simulink model "ClimberRobotModel_rbar_control"  (R2020a)
settings: Solver=VariableStepAuto  StartTime=0.0  StopTime=10.0  RelTol=1e-3
settings Model: Creator=danielefontanelli  LastModifiedBy=danielefontanelli

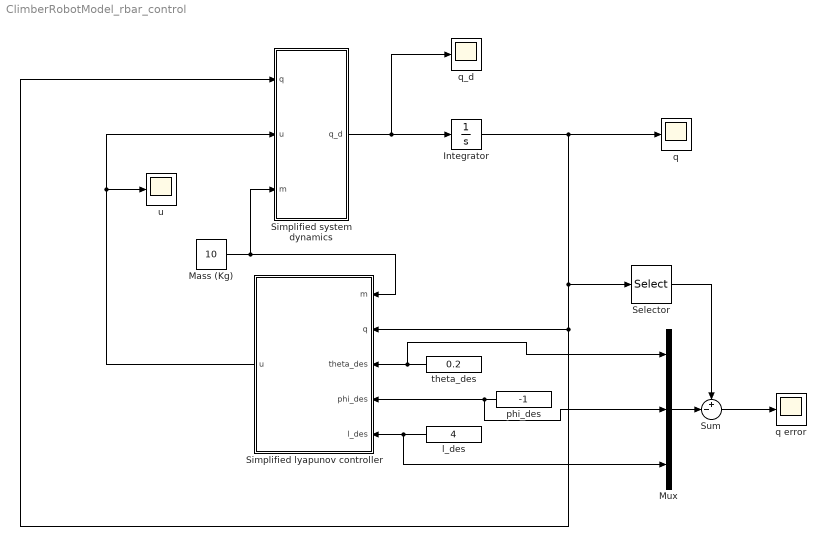
== system ClimberRobotModel_rbar_control ==
  Integrator : Integrator  InitialCondition=[0.2, -0.4, 7, 1, -1, 0]
  Mass (Kg) : Constant  Value=10
  Mux : Mux  Inputs=3
  Selector : Selector  InputPortWidth=6  IndexOptions=Index vector (dialog)  Indices=[1 2 3]  OutputSizes=1
  Simplified lyapunov controller : MATLAB Function  TreatAsAtomicUnit=on
  Simplified system dynamics : MATLAB Function  TreatAsAtomicUnit=on
  Sum : Sum  Inputs=+-|
  l_des : Constant  Value=4
  phi_des : Constant  Value=-1
  q : Scope
  q error : Scope
  q_d : Scope
  theta_des : Constant  Value=0.2
  u : Scope
  wires:
  Mass (Kg)/1 -> Simplified lyapunov controller/1(m), Simplified system dynamics/3(m)
  Simplified system dynamics/1(q_d) -> q_d/1, Integrator/1
  Integrator/1 -> q/1, Simplified system dynamics/1(q), Simplified lyapunov controller/2(q), Selector/1
  Simplified lyapunov controller/1(u) -> u/1, Simplified system dynamics/2(u)
  theta_des/1 -> Mux/1, Simplified lyapunov controller/3(theta_des)
  phi_des/1 -> Mux/2, Simplified lyapunov controller/4(phi_des)
  l_des/1 -> Mux/3, Simplified lyapunov controller/5(l_des)
  Selector/1 -> Sum/1
  Mux/1 -> Sum/2
  Sum/1 -> q error/1

== matlab function ClimberRobotModel_rbar_control/Simplified lyapunov controller ==
  data: m input; q input; u output; theta_des input; phi_des input; l_des input
function u = fcn(m, q, theta_des, phi_des, l_des)

g = 9.8;   % m/s^2

% Gains
k_theta = 1;
k_phi = 1;
k_l = 1;
k_omega = 1;
k_psi = 1;
k_r = 1;

% State space variables
theta = q(1);
phi = q(2);
l = q(3);
omega = q(4);
psi = q(5);
r = q(6);

if abs(l - l_des) < 1e-2
    Fr = 0;%sign(l - l_des);
else
    % Desired trajectories
    omega_des = -k_theta*(theta - theta_des);
    psi_des = -k_phi*(phi - phi_des);
    
    % Value of the nonlinear dynamics
    f4 = - 2*omega*r/l + psi^2*sin(theta)*cos(theta) - g/l*sin(theta);
    f5 = - 2*psi*r/l - 2*psi*omega*cos(theta)/sin(theta);
    f6 = l*(omega^2 + psi^2*sin(theta)^2) + g*cos(theta);
    
    % Desired velocities and derivatives
    omega_des_d = -k_theta*omega;
    psi_des_d = -k_phi*psi;
    h1 = (omega - omega_des)*(f4 - omega_des_d);
    h2 = (psi - psi_des)*(f5 - psi_des_d);
    h = h1 + h2;
    r_des = - h/(l - l_des) - k_l*(l - l_des)*cos(atan(h)) - k_omega*h1^2/(l - l_des) - k_psi*h2^2/(l - l_des);
    
    f4_d = (l*(2*cos(theta)^2 - 1)*psi^2 - g*cos(theta))/l*omega + (2*omega*r + g*sin(theta))/l^2*r - 2*r/l*f4 + psi*sin(2*theta)*f5 - 2*omega/l*f6;
    omega_des_dd = -k_theta*f4;
    
    f5_d = 2*omega*psi/sin(theta)^2*omega + 2*psi*r/l^2*r - 2*psi*cos(theta)/sin(theta)*f4 - (2*r/l + 2*omega*cos(theta)/sin(theta))*f5 - 2*psi/l*f6;
    psi_des_dd = -k_psi*f5;
    
    h1_d = (f4 - omega_des_d)*(f4 - omega_des_d) + (omega - omega_des)*(f4_d - omega_des_dd);
    h2_d = (f5 - psi_des_d)*(f5 - psi_des_d) + (psi - psi_des)*(f5_d - psi_des_dd);
    h_d = h1_d + h2_d;
    
    r_des_d = - (h_d - r*h)/(l - l_des)^2 - k_l*r*cos(atan(h)) + k_l*(l - l_des)*h*h_d/(h^2 + 1)^(3/2) - k_omega*(2*h1*h1_d*(l - l_des) - r*h1^2)/(l - l_des)^2 - k_psi*(2*h2*h2_d*(l - l_des) - h2^2*r)/(l - l_des)^2;
    
    % Control laws
    Fr = -m*(f6 + k_r*(r - r_des) - r_des_d);
    
    if abs(Fr) > 1e5
        aaa = 10;
    end
end

% Controls
u = Fr;

== matlab function ClimberRobotModel_rbar_control/Simplified system dynamics ==
  data: q input; u input; m input; q_d output
function q_d = fcn(q, u, m)

g = 9.8;   % m/s^2

% Inputs
Fr = u(1);

% State space variables
theta = q(1);
phi = q(2);
l = q(3);
omega = q(4);
psi = q(5);
r = q(6);

% Dynamics
theta_p = omega;
phi_p = psi;
l_p = r;
omega_p = - 2*omega*r/l + psi^2*sin(theta)*cos(theta) - g/l*sin(theta);
psi_p = - 2*psi*r/l - 2*psi*omega*cos(theta)/sin(theta);
r_p = l*(omega^2 + psi^2*sin(theta)^2) + g*cos(theta) + Fr/m;

% Outputs
q_d = [theta_p, phi_p, l_p, omega_p, psi_p, r_p]';
